simulink model "ctrl_TT"  (R2022b)
settings: Solver=FixedStepAuto  StartTime=0.0  StopTime=Tf  FixedStep=0.05  RelTol=1e-3
InitFcn:
  | run;
StopFcn:
  | save('testdata')
undefined symbols (not defined in the file): Ba_0, Bb, Bv_0, Bx_0, Cp, Cp_prime, d, dA_BP1, dA_BP2, dA_Hull, dA_PH, dA_Sail, dA_SProot, dA_X1a, dA_X1b, dA_X2a, dA_X2b, dA_X3a, dA_X3b, dA_X4a, dA_X4b, Ixx, Ixy, Ixz, Iyy, Iyz, Izz, Mb, n_BP1, n_BP2, n_Hull, n_PH, n_Sail, n_SProot, n_X2a, n_X2b, n_X3a, n_X4a, n_X4b, nt_BP1, nt_BP2, nt_Hull, nt_PH, nt_Sail, nt_SProot, nt_X1a, nt_X1b, nt_X2a, nt_X2b, nt_X3a, nt_X3b, nt_X4a, nt_X4b, Seastate, Tf, vt1_BP1, vt1_BP2, vt1_Hull, vt1_PH, vt1_Sail ... (+44)
libraries: simulink x8, sharedtransform x2, dspmathops x2
(part 3 of 5)

== system ctrl_TT/HDM/HDM B3/Z/ZdXi ==
  dX : Inport
  z : Inport  Port=2
  Demux6 : Demux  Outputs=5
  Mux : Mux  Inputs=5
  ZudX1 q+10 : Lookup_n-D  BreakpointsForDimension1=[-30 -20 -10 0 10 20 30]  BreakpointsForDimension2=[-35.0624 -15.3724 -13.8724]  BreakpointsForDimension3=[-35.0624 -15.3724 -13.8724]  Table=|  InternalRulePriority=Speed  RndMeth=Simplest
      | reshape([-0.003226964
      | -0.002116041
      | -0.001005119
      | 0.000105803
      | 0.001216725
      | 0.002327647
      | 0.003438569
      | -0.003036597
      | -0.001876165
      | -0.000715732
      | 0.0004447
      | 0.001605132
      | 0.002765565
      | 0.003925997
      | -0.003676642
      | -0.002490275
      | -0.001303908
      | -0.000117541
      | 0.001068826
      | 0.002255193
      | 0.00344156],[7,3])
      settings: InputPortMap=u0,u1
  ZudX1 q+6 : Lookup_n-D  BreakpointsForDimension1=[-30 -20 -10 0 10 20 30]  BreakpointsForDimension2=[-35.0624 -15.3724 -13.8724]  BreakpointsForDimension3=[-5.14444 -3.08666664 -1.54332]  Table=|  InternalRulePriority=Speed  RndMeth=Simplest
      | reshape([-0.001383757
      | -0.000911
      | -0.000438243
      | 3.45135E-05
      | 0.00050727
      | 0.000980027
      | 0.001452784
      | -0.001383757
      | -0.000911
      | -0.000438243
      | 3.45135E-05
      | 0.00050727
      | 0.000980027
      | 0.001452784
      | -0.001353354
      | -0.000887631
      | -0.000421908
      | 4.38143E-05
      | 0.000509537
      | 0.00097526
      | 0.001440982],[7,3])
      settings: InputPortMap=u0,u1
  ZudX1 q+7 : Lookup_n-D  BreakpointsForDimension1=[-30 -20 -10 0 10 20 30]  BreakpointsForDimension2=[-35.0624 -15.3724 -13.8724]  BreakpointsForDimension3=[-5.14444 -3.08666664 -1.54332]  Table=|  InternalRulePriority=Speed  RndMeth=Simplest
      | reshape([-0.001358511
      | -0.00091651
      | -0.000474508
      | -3.25062E-05
      | 0.000409495
      | 0.000851497
      | 0.001293499
      | -0.001303275
      | -0.00086798
      | -0.000432686
      | 2.60877E-06
      | 0.000437903
      | 0.000873198
      | 0.001308493
      | -0.001263287
      | -0.000836064
      | -0.00040884
      | 1.83841E-05
      | 0.000445608
      | 0.000872832
      | 0.001300056],[7,3])
      settings: InputPortMap=u0,u1
  ZudX1 q+8 : Lookup_n-D  BreakpointsForDimension1=[-30 -20 -10 0 10 20 30]  BreakpointsForDimension2=[-35.0624 -15.3724 -13.8724]  BreakpointsForDimension3=[-5.14444 -3.08666664 -1.54332]  Table=|  InternalRulePriority=Speed  RndMeth=Simplest
      | reshape([0.001309084
      | 0.000864124
      | 0.000419163
      | -2.5798E-05
      | -0.000470759
      | -0.000915719
      | -0.00136068
      | 0.001321953
      | 0.000882434
      | 0.000442915
      | 3.39516E-06
      | -0.000436124
      | -0.000875644
      | -0.001315163
      | 0.001313186
      | 0.000881448
      | 0.000449709
      | 1.79712E-05
      | -0.000413767
      | -0.000845505
      | -0.001277243],[7,3])
      settings: InputPortMap=u0,u1
  ZudX1 q+9 : Lookup_n-D  BreakpointsForDimension1=[-30 -20 -10 0 10 20 30]  BreakpointsForDimension2=[-35.0624 -15.3724 -13.8724]  BreakpointsForDimension3=[-5.14444 -3.08666664 -1.54332]  Table=|  InternalRulePriority=Speed  RndMeth=Simplest
      | reshape([0.001464336
      | 0.000977857
      | 0.000491377
      | 4.89775E-06
      | -0.000481582
      | -0.000968061
      | -0.00145454
      | 0.001455937
      | 0.00098192
      | 0.000507903
      | 3.38863E-05
      | -0.00044013
      | -0.000914147
      | -0.001388164
      | 0.001460604
      | 0.00098818
      | 0.000515756
      | 4.33325E-05
      | -0.000429091
      | -0.000901515
      | -0.001373939],[7,3])
      settings: InputPortMap=u0,u1
  ZdX : Outport
  wires:
  Demux6/3 -> ZudX1 q+8/1
  dX/1 -> Demux6/1
  Demux6/4 -> ZudX1 q+9/1
  Demux6/2 -> ZudX1 q+7/1
  Demux6/1 -> ZudX1 q+6/1
  Mux/1 -> ZdX/1
  Demux6/5 -> ZudX1 q+10/1
  z/1 -> ZudX1 q+6/2, ZudX1 q+7/2, ZudX1 q+8/2, ZudX1 q+10/2, ZudX1 q+9/2
  ZudX1 q+10/1 -> Mux/5
  ZudX1 q+6/1 -> Mux/1
  ZudX1 q+7/1 -> Mux/2
  ZudX1 q+8/1 -> Mux/3
  ZudX1 q+9/1 -> Mux/4

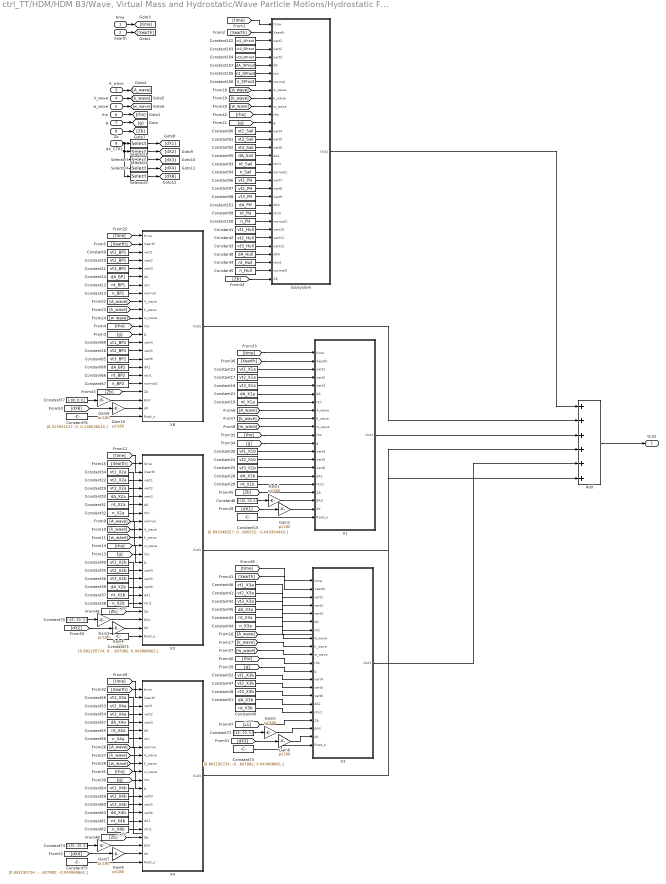
== system ctrl_TT/HDM/HDM B3/Wave, Virtual Mass and Hydrostatic/Wave Particle Motions/Hydrostatic Forces and Moments ==
  note: n_BP
  note: n_BP
  note: n_BP
  time : Inport
  Xearth : Inport  Port=2
  A_wave : Inport  Port=3
  k_wave : Inport  Port=4
  w_wave : Inport  Port=5
  rho : Inport  Port=6
  g : Inport  Port=7
  Zb : Inport  Port=8
  dX_CTRL : Inport  Port=9
  Add : Sum  Inputs=6
  Constant1 : Constant  Value=vt1_Hull
  Constant10 : Constant  Value=vt2_BP1
  Constant100 : Constant  Value=n_PH
  Constant101 : Constant  Value=dA_PH
  Constant102 : Constant  Value=vt1_SProot
  Constant103 : Constant  Value=vt2_SProot
  Constant104 : Constant  Value=vt3_SProot
  Constant105 : Constant  Value=nt_SProot
  Constant106 : Constant  Value=n_SProot
  Constant107 : Constant  Value=dA_SProot
  Constant11 : Constant  Value=vt3_BP1
  Constant12 : Constant  Value=nt_BP1
  Constant13 : Constant  Value=n_BP1
  Constant14 : Constant  Value=dA_BP1
  Constant15 : Constant  Value=|
      | [0.893348257;
      | 0.043600552;
      | -0.043394945;]
  Constant16 : Constant  Value=vt2_BP2
  Constant17 : Constant  Value=vt2_X1a
  Constant18 : Constant  Value=vt3_X1a
  Constant19 : Constant  Value=nt_X1a
  Constant2 : Constant  Value=vt2_Hull
  Constant21 : Constant  Value=dA_X1a
  Constant22 : Constant  Value=vt2_X2a
  Constant23 : Constant  Value=vt1_X1a
  Constant24 : Constant  Value=vt2_X1b
  Constant25 : Constant  Value=vt3_X1b
  Constant26 : Constant  Value=nt_X1b
  Constant28 : Constant  Value=dA_X1b
  Constant29 : Constant  Value=vt3_X2a
  Constant3 : Constant  Value=vt3_Hull
  Constant30 : Constant  Value=vt1_X1b
  Constant31 : Constant  Value=nt_X2a
  Constant32 : Constant  Value=n_X2a
  Constant33 : Constant  Value=dA_X2a
  Constant34 : Constant  Value=vt1_X2a
  Constant35 : Constant  Value=vt2_X2b
  Constant36 : Constant  Value=vt3_X2b
  Constant37 : Constant  Value=nt_X2b
  Constant38 : Constant  Value=n_X2b
  Constant39 : Constant  Value=dA_X2b
  Constant4 : Constant  Value=nt_Hull
  Constant40 : Constant  Value=vt1_X2b
  Constant41 : Constant  Value=vt2_X3a
  Constant42 : Constant  Value=vt3_X3a
  Constant43 : Constant  Value=nt_X3a
  Constant44 : Constant  Value=n_X3a
  Constant45 : Constant  Value=dA_X3a
  Constant46 : Constant  Value=vt1_X3a
  Constant47 : Constant  Value=vt2_X3b
  Constant48 : Constant  Value=vt3_X3b
  Constant49 : Constant  Value=nt_X3b
  Constant5 : Constant  Value=n_Hull
  Constant51 : Constant  Value=dA_X3b
  Constant52 : Constant  Value=vt1_X3b
  Constant53 : Constant  Value=vt2_X4a
  Constant54 : Constant  Value=vt3_X4a
  Constant55 : Constant  Value=nt_X4a
  Constant56 : Constant  Value=n_X4a
  Constant57 : Constant  Value=dA_X4a
  Constant58 : Constant  Value=vt1_X4a
  Constant59 : Constant  Value=vt2_X4b
  Constant6 : Constant  Value=[-135; -20; 0;]
  Constant60 : Constant  Value=vt3_X4b
  Constant61 : Constant  Value=nt_X4b
  Constant62 : Constant  Value=n_X4b
  Constant63 : Constant  Value=dA_X4b
  Constant64 : Constant  Value=vt1_X4b
  Constant65 : Constant  Value=vt3_BP2
  Constant66 : Constant  Value=nt_BP2
  Constant67 : Constant  Value=n_BP2
  Constant68 : Constant  Value=dA_BP2
  Constant69 : Constant  Value=vt1_BP2
  Constant70 : Constant  Value=[-45; -20; 0;]
  Constant71 : Constant  Value=|
      | [0.892195724;
      | 0.043607982;
      | 0.043868661;]
  Constant72 : Constant  Value=[45; -20; 0;]
  Constant73 : Constant  Value=|
      | [0.892195724;
      | -0.043607982;
      | 0.043868661;]
  Constant74 : Constant  Value=[135; -20; 0;]
  Constant75 : Constant  Value=|
      | [0.892195724;
      | -0.043607982;
      | -0.043868661;]
  Constant76 : Constant  Value=|
      | [0.313941517;
      | 0;
      | 0.138536015;]
  Constant77 : Constant  Value=[-90; 0; 0;]
  Constant8 : Constant  Value=dA_Hull
  Constant9 : Constant  Value=vt1_BP1
  Constant90 : Constant  Value=vt1_Sail
  Constant91 : Constant  Value=vt2_Sail
  Constant92 : Constant  Value=vt3_Sail
  Constant93 : Constant  Value=nt_Sail
  Constant94 : Constant  Value=n_Sail
  Constant95 : Constant  Value=dA_Sail
  Constant96 : Constant  Value=vt1_PH
  Constant97 : Constant  Value=vt2_PH
  Constant98 : Constant  Value=vt3_PH
  Constant99 : Constant  Value=nt_PH
  Gain{1..10} (10 alike) : Gain  Gain=pi/180
  Selector1 : Selector  InputPortWidth=5  IndexOptions=Index vector (dialog)  Indices=1  OutputSizes=1
  Selector2 : Selector  InputPortWidth=5  IndexOptions=Index vector (dialog)  Indices=2  OutputSizes=1
  Selector3 : Selector  InputPortWidth=5  IndexOptions=Index vector (dialog)  Indices=3  OutputSizes=1
  Selector4 : Selector  InputPortWidth=5  IndexOptions=Index vector (dialog)  Indices=4  OutputSizes=1
  Selector5 : Selector  InputPortWidth=5  IndexOptions=Index vector (dialog)  Indices=5  OutputSizes=1
  Subsystem : Subsystem
  X1 : Subsystem
  X2 : Subsystem
  X3 : Subsystem
  X4 : Subsystem
  XB : Subsystem
  Out1 : Outport
  wires:
  Subsystem/1(Out1) -> Add/1
  XB/1(Out1) -> Add/2
  X1/1(Out1) -> Add/3
  X2/1(Out1) -> Add/4
  X3/1(Out1) -> Add/5
  X4/1(Out1) -> Add/6
  Gain10/1 -> XB/22(dX)
  Constant76/1 -> XB/23(Root_o)
  [dXB] -> Gain10/1
  Gain9/1 -> XB/21(EAX)
  Constant77/1 -> Gain9/1
  Gain8/1 -> X4/21(dX)
  [dX4] -> Gain8/1
  Constant74/1 -> Gain7/1
  Gain7/1 -> X4/20(EAX)
  Constant75/1 -> X4/22(Root_o)
  Constant73/1 -> X3/21(Root_o)
  Gain6/1 -> X3/20(dX)
  Constant72/1 -> Gain5/1
  [dX3] -> Gain6/1
  Gain5/1 -> X3/19(EAX)
  Constant71/1 -> X2/22(Root_o)
  Gain4/1 -> X2/21(dX)
  [dX2] -> Gain4/1
  Gain3/1 -> X2/20(EAX)
  Constant70/1 -> Gain3/1
  Constant15/1 -> X1/21(Root_o)
  Gain2/1 -> X1/20(dX)
  [dX1] -> Gain2/1
  Selector5/1 -> [dXB]
  Selector4/1 -> [dX4]
  Selector3/1 -> [dX3]
  Selector2/1 -> [dX2]
  Selector1/1 -> [dX1]
  dX_CTRL/1 -> Selector1/1, Selector4/1, Selector5/1, Selector3/1, Selector2/1
  Gain1/1 -> X1/19(EAX)
  Constant6/1 -> Gain1/1
  Zb/1 -> [Zb]
  [A_wave] -> X3/8(A_wave)
  Constant5/1 -> Subsystem/31(normal3)
  Constant58/1 -> X4/3(vert1)
  Constant42/1 -> X3/5(vert3)
  [g] -> XB/13(g)
  Constant3/1 -> Subsystem/28(vert12)
  Constant103/1 -> Subsystem/4(vert2)
  Add/1 -> Out1/1
  [A_wave] -> Subsystem/9(A_wave)
  Constant10/1 -> XB/4(vert2)
  [time] -> X4/1(time)
  [k_wave] -> X4/10(k_wave)
  Constant38/1 -> ?
  Constant54/1 -> X4/5(vert3)
  Constant66/1 -> XB/18(ntri1)
  Constant2/1 -> Subsystem/27(vert11)
  Constant97/1 -> Subsystem/21(vert8)
  Constant64/1 -> X4/14(vert4)
  [Xearth] -> X4/2(Xearth)
  Constant29/1 -> X2/5(vert3)
  Constant36/1 -> X2/16(vert6)
  Constant96/1 -> Subsystem/20(vert7)
  Constant90/1 -> Subsystem/14(vert4)
  Constant21/1 -> X1/6(dA)
  [w_wave] -> X2/11(w_wave)
  Constant31/1 -> X2/7(ntri)
  Constant1/1 -> Subsystem/26(vert10)
  [time] -> X1/1(time)
  Constant91/1 -> Subsystem/15(vert5)
  [rho] -> X1/11(rho)
  [time] -> X2/1(time)
  Constant30/1 -> X1/13(vert4)
  Constant92/1 -> Subsystem/16(vert6)
  Constant100/1 -> Subsystem/25(normal2)
  [w_wave] -> X1/10(w_wave)
  [g] -> X3/12(g)
  Constant12/1 -> XB/7(ntri)
  Constant24/1 -> X1/14(vert5)
  Constant56/1 -> X4/8(normal)
  Constant26/1 -> X1/17(ntri1)
  [A_wave] -> XB/9(A_wave)
  Constant62/1 -> ?
  Constant9/1 -> XB/3(vert1)
  Constant23/1 -> X1/3(vert1)
  Constant46/1 -> X3/3(vert1)
  Constant68/1 -> XB/17(dA1)
  [k_wave] -> XB/10(k_wave)
  Constant17/1 -> X1/4(vert2)
  [A_wave] -> X2/9(A_wave)
  [k_wave] -> X3/9(k_wave)
  Constant43/1 -> X3/7(ntri)
  Constant69/1 -> XB/14(vert4)
  Constant13/1 -> XB/8(normal)
  Constant104/1 -> Subsystem/5(vert3)
  Constant65/1 -> XB/16(vert6)
  [Zb] -> Subsystem/32(Zb)
  Constant67/1 -> XB/19(normal1)
  Constant25/1 -> X1/15(vert6)
  [Xearth] -> X3/2(Xearth)
  Constant14/1 -> XB/6(dA)
  Constant52/1 -> X3/13(vert4)
  Constant51/1 -> X3/16(dA1)
  Constant59/1 -> X4/15(vert5)
  Constant4/1 -> Subsystem/30(ntri3)
  [rho] -> XB/12(rho)
  [time] -> XB/1(time)
  [Xearth] -> X2/2(Xearth)
  [w_wave] -> XB/11(w_wave)
  Constant53/1 -> X4/4(vert2)
  [k_wave] -> X1/9(k_wave)
  Constant44/1 -> ?
  [w_wave] -> X4/11(w_wave)
  Constant47/1 -> X3/14(vert5)
  Constant32/1 -> X2/8(normal)
  Constant39/1 -> X2/17(dA1)
  Constant35/1 -> X2/15(vert5)
  [g] -> X1/12(g)
  Constant18/1 -> X1/5(vert3)
  Constant40/1 -> X2/14(vert4)
  Constant45/1 -> X3/6(dA)
  Constant55/1 -> X4/7(ntri)
  [rho] -> X3/11(rho)
  [rho] -> X2/12(rho)
  [Xearth] -> XB/2(Xearth)
  Constant49/1 -> X3/17(ntri1)
  Constant22/1 -> X2/4(vert2)
  [k_wave] -> X2/10(k_wave)
  Constant41/1 -> X3/4(vert2)
  [A_wave] -> X1/8(A_wave)
  Constant63/1 -> X4/17(dA1)
  Constant34/1 -> X2/3(vert1)
  Constant11/1 -> XB/5(vert3)
  [g] -> X4/13(g)
  Constant105/1 -> Subsystem/7(ntri)
  Constant107/1 -> Subsystem/6(dA)
  [Xearth] -> Subsystem/2(Xearth)
  Constant106/1 -> Subsystem/8(normal)
  Constant102/1 -> Subsystem/3(vert1)
  [g] -> Subsystem/13(g)
  Constant19/1 -> X1/7(ntri)
  [k_wave] -> Subsystem/10(k_wave)
  Constant60/1 -> X4/16(vert6)
  [rho] -> Subsystem/12(rho)
  Constant48/1 -> X3/15(vert6)
  [time] -> Subsystem/1(time)
  [rho] -> X4/12(rho)
  Constant33/1 -> X2/6(dA)
  [A_wave] -> X4/9(A_wave)
  Constant95/1 -> Subsystem/17(dA1)
  Constant8/1 -> Subsystem/29(dA3)
  [w_wave] -> X3/10(w_wave)
  Constant28/1 -> X1/16(dA1)
  [g] -> X2/13(g)
  Constant93/1 -> Subsystem/18(ntri1)
  [w_wave] -> Subsystem/11(w_wave)
  [Xearth] -> X1/2(Xearth)
  [time] -> X3/1(time)
  [Zb] -> XB/20(Zb)
  Constant37/1 -> X2/18(ntri1)
  Constant99/1 -> Subsystem/24(ntri2)
  Constant98/1 -> Subsystem/22(vert9)
  [Zb] -> X2/19(Zb)
  [Zb] -> X1/18(Zb)
  Constant16/1 -> XB/15(vert5)
  Constant101/1 -> Subsystem/23(dA2)
  [Zb] -> X3/18(Zb)
  [Zb] -> X4/19(Zb)
  Constant57/1 -> X4/6(dA)
  Constant61/1 -> X4/18(ntri1)
  Constant94/1 -> Subsystem/19(normal1)
  g/1 -> [g]
  rho/1 -> [rho]
  w_wave/1 -> [w_wave]
  k_wave/1 -> [k_wave]
  A_wave/1 -> [A_wave]
  Xearth/1 -> [Xearth]
  time/1 -> [time]

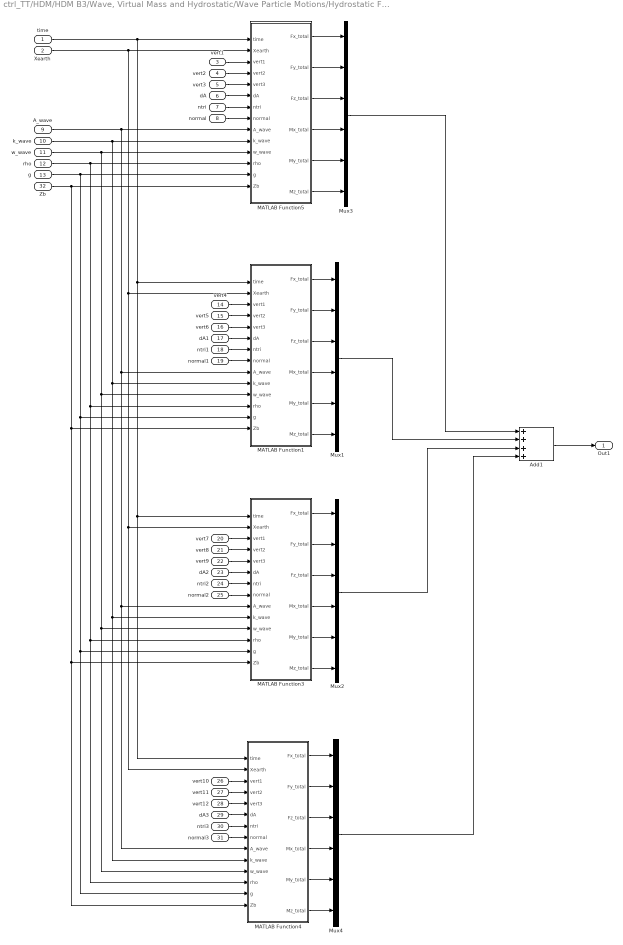
== system ctrl_TT/HDM/HDM B3/Wave, Virtual Mass and Hydrostatic/Wave Particle Motions/Hydrostatic Forces and Moments/Subsystem ==
  time : Inport
  Xearth : Inport  Port=2
  vert1 : Inport  Port=3
  vert2 : Inport  Port=4
  vert3 : Inport  Port=5
  dA : Inport  Port=6
  ntri : Inport  Port=7
  normal : Inport  Port=8
  A_wave : Inport  Port=9
  k_wave : Inport  Port=10
  w_wave : Inport  Port=11
  rho : Inport  Port=12
  g : Inport  Port=13
  vert4 : Inport  Port=14
  vert5 : Inport  Port=15
  vert6 : Inport  Port=16
  dA1 : Inport  Port=17
  ntri1 : Inport  Port=18
  normal1 : Inport  Port=19
  vert7 : Inport  Port=20
  vert8 : Inport  Port=21
  vert9 : Inport  Port=22
  dA2 : Inport  Port=23
  ntri2 : Inport  Port=24
  normal2 : Inport  Port=25
  vert10 : Inport  Port=26
  vert11 : Inport  Port=27
  vert12 : Inport  Port=28
  dA3 : Inport  Port=29
  ntri3 : Inport  Port=30
  normal3 : Inport  Port=31
  Zb : Inport  Port=32
  Add1 : Sum  Inputs=4
  MATLAB Function1 : MATLAB Function  TreatAsAtomicUnit=on
  MATLAB Function3 : MATLAB Function  TreatAsAtomicUnit=on
  MATLAB Function4 : MATLAB Function  TreatAsAtomicUnit=on
  MATLAB Function5 : MATLAB Function  TreatAsAtomicUnit=on
  Mux{1..4} (4 alike) : Mux  Inputs=6
  Out1 : Outport
  wires:
  Mux4/1 -> Add1/4
  MATLAB Function4/5(My_total) -> Mux4/5
  MATLAB Function4/4(Mx_total) -> Mux4/4
  MATLAB Function4/3(Fz_total) -> Mux4/3
  MATLAB Function4/2(Fy_total) -> Mux4/2
  MATLAB Function4/1(Fx_total) -> Mux4/1
  MATLAB Function4/6(Mz_total) -> Mux4/6
  MATLAB Function3/6(Mz_total) -> Mux2/6
  MATLAB Function3/1(Fx_total) -> Mux2/1
  MATLAB Function3/2(Fy_total) -> Mux2/2
  MATLAB Function3/3(Fz_total) -> Mux2/3
  MATLAB Function3/4(Mx_total) -> Mux2/4
  MATLAB Function3/5(My_total) -> Mux2/5
  MATLAB Function1/5(My_total) -> Mux1/5
  MATLAB Function1/4(Mx_total) -> Mux1/4
  MATLAB Function1/3(Fz_total) -> Mux1/3
  MATLAB Function1/2(Fy_total) -> Mux1/2
  MATLAB Function1/1(Fx_total) -> Mux1/1
  Mux1/1 -> Add1/2
  MATLAB Function1/6(Mz_total) -> Mux1/6
  Mux2/1 -> Add1/3
  Zb/1 -> MATLAB Function4/14(Zb), MATLAB Function3/14(Zb), MATLAB Function1/14(Zb), MATLAB Function5/14(Zb)
  vert8/1 -> MATLAB Function3/4(vert2)
  vert1/1 -> MATLAB Function5/3(vert1)
  vert10/1 -> MATLAB Function4/3(vert1)
  dA1/1 -> MATLAB Function1/6(dA)
  normal2/1 -> MATLAB Function3/8(normal)
  vert3/1 -> MATLAB Function5/5(vert3)
  vert6/1 -> MATLAB Function1/5(vert3)
  Add1/1 -> Out1/1
  vert2/1 -> MATLAB Function5/4(vert2)
  dA3/1 -> MATLAB Function4/6(dA)
  ntri3/1 -> MATLAB Function4/7(ntri)
  ntri2/1 -> MATLAB Function3/7(ntri)
  vert11/1 -> MATLAB Function4/4(vert2)
  MATLAB Function5/6(Mz_total) -> Mux3/6
  dA/1 -> MATLAB Function5/6(dA)
  normal/1 -> MATLAB Function5/8(normal)
  vert9/1 -> MATLAB Function3/5(vert3)
  vert4/1 -> MATLAB Function1/3(vert1)
  normal3/1 -> MATLAB Function4/8(normal)
  vert12/1 -> MATLAB Function4/5(vert3)
  MATLAB Function5/1(Fx_total) -> Mux3/1
  dA2/1 -> MATLAB Function3/6(dA)
  g/1 -> MATLAB Function3/13(g), MATLAB Function4/13(g), MATLAB Function1/13(g), MATLAB Function5/13(g)
  ntri/1 -> MATLAB Function5/7(ntri)
  MATLAB Function5/2(Fy_total) -> Mux3/2
  w_wave/1 -> MATLAB Function3/11(w_wave), MATLAB Function4/11(w_wave), MATLAB Function1/11(w_wave), MATLAB Function5/11(w_wave)
  k_wave/1 -> MATLAB Function3/10(k_wave), MATLAB Function4/10(k_wave), MATLAB Function1/10(k_wave), MATLAB Function5/10(k_wave)
  MATLAB Function5/3(Fz_total) -> Mux3/3
  A_wave/1 -> MATLAB Function3/9(A_wave), MATLAB Function4/9(A_wave), MATLAB Function1/9(A_wave), MATLAB Function5/9(A_wave)
  normal1/1 -> MATLAB Function1/8(normal)
  Mux3/1 -> Add1/1
  MATLAB Function5/4(Mx_total) -> Mux3/4
  vert7/1 -> MATLAB Function3/3(vert1)
  Xearth/1 -> MATLAB Function1/2(Xearth), MATLAB Function3/2(Xearth), MATLAB Function4/2(Xearth), MATLAB Function5/2(Xearth)
  time/1 -> MATLAB Function3/1(time), MATLAB Function4/1(time), MATLAB Function1/1(time), MATLAB Function5/1(time)
  MATLAB Function5/5(My_total) -> Mux3/5
  vert5/1 -> MATLAB Function1/4(vert2)
  rho/1 -> MATLAB Function3/12(rho), MATLAB Function4/12(rho), MATLAB Function1/12(rho), MATLAB Function5/12(rho)
  ntri1/1 -> MATLAB Function1/7(ntri)

== system ctrl_TT/HDM/HDM B3/Wave, Virtual Mass and Hydrostatic/Wave Particle Motions/Hydrostatic Forces and Moments/X1 ==
  time : Inport
  Xearth : Inport  Port=2
  vert1 : Inport  Port=3
  vert2 : Inport  Port=4
  vert3 : Inport  Port=5
  dA : Inport  Port=6
  ntri : Inport  Port=7
  A_wave : Inport  Port=8
  k_wave : Inport  Port=9
  w_wave : Inport  Port=10
  rho : Inport  Port=11
  g : Inport  Port=12
  vert4 : Inport  Port=13
  vert5 : Inport  Port=14
  vert6 : Inport  Port=15
  dA1 : Inport  Port=16
  ntri1 : Inport  Port=17
  Zb : Inport  Port=18
  EAX : Inport  Port=19
  dX : Inport  Port=20
  Root_o : Inport  Port=21
  Add1 : Sum
  CG : Constant  Value=[32.3114; 0; 0;]
  MATLAB Function1 : MATLAB Function  TreatAsAtomicUnit=on
  MATLAB Function4 : MATLAB Function  TreatAsAtomicUnit=on
  Mux1 : Mux  Inputs=6
  Mux2 : Mux  Inputs=6
  Out1 : Outport
  wires:
  MATLAB Function1/6(Mz_total) -> Mux1/6
  MATLAB Function1/5(My_total) -> Mux1/5
  CG/1 -> MATLAB Function4/17(xcg), MATLAB Function1/17(xcg)
  Root_o/1 -> MATLAB Function4/16(origin), MATLAB Function1/16(origin)
  dX/1 -> MATLAB Function1/15(dX), MATLAB Function4/15(dX)
  EAX/1 -> MATLAB Function4/14(EAX), MATLAB Function1/14(EAX)
  MATLAB Function4/3(Fz_total) -> Mux2/3
  MATLAB Function4/4(Mx_total) -> Mux2/4
  w_wave/1 -> MATLAB Function4/10(w_wave), MATLAB Function1/10(w_wave)
  MATLAB Function1/2(Fy_total) -> Mux1/2
  Xearth/1 -> MATLAB Function1/2(Xearth), MATLAB Function4/2(Xearth)
  rho/1 -> MATLAB Function4/11(rho), MATLAB Function1/11(rho)
  A_wave/1 -> MATLAB Function4/8(A_wave), MATLAB Function1/8(A_wave)
  MATLAB Function1/4(Mx_total) -> Mux1/4
  MATLAB Function4/1(Fx_total) -> Mux2/1
  MATLAB Function1/1(Fx_total) -> Mux1/1
  Add1/1 -> Out1/1
  MATLAB Function1/3(Fz_total) -> Mux1/3
  MATLAB Function4/5(My_total) -> Mux2/5
  dA/1 -> MATLAB Function4/6(dA)
  k_wave/1 -> MATLAB Function1/9(k_wave), MATLAB Function4/9(k_wave)
  g/1 -> MATLAB Function4/12(g), MATLAB Function1/12(g)
  MATLAB Function4/6(Mz_total) -> Mux2/6
  MATLAB Function4/2(Fy_total) -> Mux2/2
  Mux2/1 -> Add1/1
  vert3/1 -> MATLAB Function4/5(vert3)
  Mux1/1 -> Add1/2
  vert1/1 -> MATLAB Function4/3(vert1)
  time/1 -> MATLAB Function1/1(time), MATLAB Function4/1(time)
  ntri/1 -> MATLAB Function4/7(ntri)
  vert2/1 -> MATLAB Function4/4(vert2)
  Zb/1 -> MATLAB Function4/13(Zb), MATLAB Function1/13(Zb)
  vert4/1 -> MATLAB Function1/3(vert1)
  vert5/1 -> MATLAB Function1/4(vert2)
  vert6/1 -> MATLAB Function1/5(vert3)
  dA1/1 -> MATLAB Function1/6(dA)
  ntri1/1 -> MATLAB Function1/7(ntri)

== system ctrl_TT/HDM/HDM B3/Wave, Virtual Mass and Hydrostatic/Wave Particle Motions/Hydrostatic Forces and Moments/X2 ==
  time : Inport
  Xearth : Inport  Port=2
  vert1 : Inport  Port=3
  vert2 : Inport  Port=4
  vert3 : Inport  Port=5
  dA : Inport  Port=6
  ntri : Inport  Port=7
  normal : Inport  Port=8
  A_wave : Inport  Port=9
  k_wave : Inport  Port=10
  w_wave : Inport  Port=11
  rho : Inport  Port=12
  g : Inport  Port=13
  vert4 : Inport  Port=14
  vert5 : Inport  Port=15
  vert6 : Inport  Port=16
  dA1 : Inport  Port=17
  ntri1 : Inport  Port=18
  Zb : Inport  Port=19
  EAX : Inport  Port=20
  dX : Inport  Port=21
  Root_o : Inport  Port=22
  Add1 : Sum
  CG : Constant  Value=[32.3114; 0; 0;]
  MATLAB Function1 : MATLAB Function  TreatAsAtomicUnit=on
  MATLAB Function4 : MATLAB Function  TreatAsAtomicUnit=on
  Mux1 : Mux  Inputs=6
  Mux2 : Mux  Inputs=6
  Out1 : Outport
  wires:
  ntri1/1 -> MATLAB Function1/7(ntri)
  dA1/1 -> MATLAB Function1/6(dA)
  vert6/1 -> MATLAB Function1/5(vert3)
  vert5/1 -> MATLAB Function1/4(vert2)
  vert4/1 -> MATLAB Function1/3(vert1)
  Zb/1 -> MATLAB Function4/13(Zb), MATLAB Function1/13(Zb)
  vert2/1 -> MATLAB Function4/4(vert2)
  ntri/1 -> MATLAB Function4/7(ntri)
  normal/1 -> ?
  time/1 -> MATLAB Function4/1(time), MATLAB Function1/1(time)
  vert1/1 -> MATLAB Function4/3(vert1)
  Mux1/1 -> Add1/2
  vert3/1 -> MATLAB Function4/5(vert3)
  Mux2/1 -> Add1/1
  MATLAB Function4/2(Fy_total) -> Mux2/2
  MATLAB Function4/6(Mz_total) -> Mux2/6
  g/1 -> MATLAB Function4/12(g), MATLAB Function1/12(g)
  k_wave/1 -> MATLAB Function4/9(k_wave), MATLAB Function1/9(k_wave)
  dA/1 -> MATLAB Function4/6(dA)
  MATLAB Function4/5(My_total) -> Mux2/5
  MATLAB Function1/3(Fz_total) -> Mux1/3
  Add1/1 -> Out1/1
  MATLAB Function1/1(Fx_total) -> Mux1/1
  MATLAB Function4/1(Fx_total) -> Mux2/1
  MATLAB Function1/4(Mx_total) -> Mux1/4
  A_wave/1 -> MATLAB Function4/8(A_wave), MATLAB Function1/8(A_wave)
  rho/1 -> MATLAB Function4/11(rho), MATLAB Function1/11(rho)
  Xearth/1 -> MATLAB Function4/2(Xearth), MATLAB Function1/2(Xearth)
  MATLAB Function1/2(Fy_total) -> Mux1/2
  w_wave/1 -> MATLAB Function4/10(w_wave), MATLAB Function1/10(w_wave)
  MATLAB Function4/4(Mx_total) -> Mux2/4
  MATLAB Function4/3(Fz_total) -> Mux2/3
  EAX/1 -> MATLAB Function4/14(EAX), MATLAB Function1/14(EAX)
  dX/1 -> MATLAB Function4/15(dX), MATLAB Function1/15(dX)
  Root_o/1 -> MATLAB Function4/16(origin), MATLAB Function1/16(origin)
  CG/1 -> MATLAB Function4/17(xcg), MATLAB Function1/17(xcg)
  MATLAB Function1/5(My_total) -> Mux1/5
  MATLAB Function1/6(Mz_total) -> Mux1/6

== system ctrl_TT/HDM/HDM B3/Wave, Virtual Mass and Hydrostatic/Wave Particle Motions/Hydrostatic Forces and Moments/X3 ==
  time : Inport
  Xearth : Inport  Port=2
  vert1 : Inport  Port=3
  vert2 : Inport  Port=4
  vert3 : Inport  Port=5
  dA : Inport  Port=6
  ntri : Inport  Port=7
  A_wave : Inport  Port=8
  k_wave : Inport  Port=9
  w_wave : Inport  Port=10
  rho : Inport  Port=11
  g : Inport  Port=12
  vert4 : Inport  Port=13
  vert5 : Inport  Port=14
  vert6 : Inport  Port=15
  dA1 : Inport  Port=16
  ntri1 : Inport  Port=17
  Zb : Inport  Port=18
  EAX : Inport  Port=19
  dX : Inport  Port=20
  Root_o : Inport  Port=21
  Add1 : Sum
  CG : Constant  Value=[32.3114; 0; 0;]
  MATLAB Function1 : MATLAB Function  TreatAsAtomicUnit=on
  MATLAB Function4 : MATLAB Function  TreatAsAtomicUnit=on
  Mux1 : Mux  Inputs=6
  Mux2 : Mux  Inputs=6
  Out1 : Outport
  wires:
  MATLAB Function1/6(Mz_total) -> Mux1/6
  MATLAB Function1/5(My_total) -> Mux1/5
  CG/1 -> MATLAB Function1/17(xcg), MATLAB Function4/17(xcg)
  Root_o/1 -> MATLAB Function1/16(origin), MATLAB Function4/16(origin)
  dX/1 -> MATLAB Function1/15(dX), MATLAB Function4/15(dX)
  EAX/1 -> MATLAB Function1/14(EAX), MATLAB Function4/14(EAX)
  MATLAB Function4/3(Fz_total) -> Mux2/3
  MATLAB Function4/4(Mx_total) -> Mux2/4
  w_wave/1 -> MATLAB Function1/10(w_wave), MATLAB Function4/10(w_wave)
  MATLAB Function1/2(Fy_total) -> Mux1/2
  Xearth/1 -> MATLAB Function1/2(Xearth), MATLAB Function4/2(Xearth)
  rho/1 -> MATLAB Function1/11(rho), MATLAB Function4/11(rho)
  A_wave/1 -> MATLAB Function1/8(A_wave), MATLAB Function4/8(A_wave)
  MATLAB Function1/4(Mx_total) -> Mux1/4
  MATLAB Function4/1(Fx_total) -> Mux2/1
  MATLAB Function1/1(Fx_total) -> Mux1/1
  Add1/1 -> Out1/1
  MATLAB Function1/3(Fz_total) -> Mux1/3
  MATLAB Function4/5(My_total) -> Mux2/5
  dA/1 -> MATLAB Function4/6(dA)
  k_wave/1 -> MATLAB Function1/9(k_wave), MATLAB Function4/9(k_wave)
  g/1 -> MATLAB Function1/12(g), MATLAB Function4/12(g)
  MATLAB Function4/6(Mz_total) -> Mux2/6
  MATLAB Function4/2(Fy_total) -> Mux2/2
  Mux2/1 -> Add1/1
  vert3/1 -> MATLAB Function4/5(vert3)
  Mux1/1 -> Add1/2
  vert1/1 -> MATLAB Function4/3(vert1)
  time/1 -> MATLAB Function1/1(time), MATLAB Function4/1(time)
  ntri/1 -> MATLAB Function4/7(ntri)
  vert2/1 -> MATLAB Function4/4(vert2)
  Zb/1 -> MATLAB Function1/13(Zb), MATLAB Function4/13(Zb)
  vert4/1 -> MATLAB Function1/3(vert1)
  vert5/1 -> MATLAB Function1/4(vert2)
  vert6/1 -> MATLAB Function1/5(vert3)
  dA1/1 -> MATLAB Function1/6(dA)
  ntri1/1 -> MATLAB Function1/7(ntri)

== system ctrl_TT/HDM/HDM B3/Wave, Virtual Mass and Hydrostatic/Wave Particle Motions/Hydrostatic Forces and Moments/X4 ==
  time : Inport
  Xearth : Inport  Port=2
  vert1 : Inport  Port=3
  vert2 : Inport  Port=4
  vert3 : Inport  Port=5
  dA : Inport  Port=6
  ntri : Inport  Port=7
  normal : Inport  Port=8
  A_wave : Inport  Port=9
  k_wave : Inport  Port=10
  w_wave : Inport  Port=11
  rho : Inport  Port=12
  g : Inport  Port=13
  vert4 : Inport  Port=14
  vert5 : Inport  Port=15
  vert6 : Inport  Port=16
  dA1 : Inport  Port=17
  ntri1 : Inport  Port=18
  Zb : Inport  Port=19
  EAX : Inport  Port=20
  dX : Inport  Port=21
  Root_o : Inport  Port=22
  Add1 : Sum
  CG : Constant  Value=[32.3114; 0; 0;]
  MATLAB Function1 : MATLAB Function  TreatAsAtomicUnit=on
  MATLAB Function4 : MATLAB Function  TreatAsAtomicUnit=on
  Mux1 : Mux  Inputs=6
  Mux2 : Mux  Inputs=6
  Out1 : Outport
  wires:
  ntri1/1 -> MATLAB Function1/7(ntri)
  dA1/1 -> MATLAB Function1/6(dA)
  vert6/1 -> MATLAB Function1/5(vert3)
  vert5/1 -> MATLAB Function1/4(vert2)
  vert4/1 -> MATLAB Function1/3(vert1)
  Zb/1 -> MATLAB Function4/13(Zb), MATLAB Function1/13(Zb)
  vert2/1 -> MATLAB Function4/4(vert2)
  ntri/1 -> MATLAB Function4/7(ntri)
  normal/1 -> ?
  time/1 -> MATLAB Function4/1(time), MATLAB Function1/1(time)
  vert1/1 -> MATLAB Function4/3(vert1)
  Mux1/1 -> Add1/2
  vert3/1 -> MATLAB Function4/5(vert3)
  Mux2/1 -> Add1/1
  MATLAB Function4/2(Fy_total) -> Mux2/2
  MATLAB Function4/6(Mz_total) -> Mux2/6
  g/1 -> MATLAB Function4/12(g), MATLAB Function1/12(g)
  k_wave/1 -> MATLAB Function4/9(k_wave), MATLAB Function1/9(k_wave)
  dA/1 -> MATLAB Function4/6(dA)
  MATLAB Function4/5(My_total) -> Mux2/5
  MATLAB Function1/3(Fz_total) -> Mux1/3
  Add1/1 -> Out1/1
  MATLAB Function1/1(Fx_total) -> Mux1/1
  MATLAB Function4/1(Fx_total) -> Mux2/1
  MATLAB Function1/4(Mx_total) -> Mux1/4
  A_wave/1 -> MATLAB Function4/8(A_wave), MATLAB Function1/8(A_wave)
  rho/1 -> MATLAB Function1/11(rho), MATLAB Function4/11(rho)
  Xearth/1 -> MATLAB Function4/2(Xearth), MATLAB Function1/2(Xearth)
  MATLAB Function1/2(Fy_total) -> Mux1/2
  w_wave/1 -> MATLAB Function4/10(w_wave), MATLAB Function1/10(w_wave)
  MATLAB Function4/4(Mx_total) -> Mux2/4
  MATLAB Function4/3(Fz_total) -> Mux2/3
  EAX/1 -> MATLAB Function4/14(EAX), MATLAB Function1/14(EAX)
  dX/1 -> MATLAB Function4/15(dX), MATLAB Function1/15(dX)
  Root_o/1 -> MATLAB Function4/16(origin), MATLAB Function1/16(origin)
  CG/1 -> MATLAB Function4/17(xcg), MATLAB Function1/17(xcg)
  MATLAB Function1/5(My_total) -> Mux1/5
  MATLAB Function1/6(Mz_total) -> Mux1/6

== system ctrl_TT/HDM/HDM B3/Wave, Virtual Mass and Hydrostatic/Wave Particle Motions/Hydrostatic Forces and Moments/XB ==
  time : Inport
  Xearth : Inport  Port=2
  vert1 : Inport  Port=3
  vert2 : Inport  Port=4
  vert3 : Inport  Port=5
  dA : Inport  Port=6
  ntri : Inport  Port=7
  normal : Inport  Port=8
  A_wave : Inport  Port=9
  k_wave : Inport  Port=10
  w_wave : Inport  Port=11
  rho : Inport  Port=12
  g : Inport  Port=13
  vert4 : Inport  Port=14
  vert5 : Inport  Port=15
  vert6 : Inport  Port=16
  dA1 : Inport  Port=17
  ntri1 : Inport  Port=18
  normal1 : Inport  Port=19
  Zb : Inport  Port=20
  EAX : Inport  Port=21
  dX : Inport  Port=22
  Root_o : Inport  Port=23
  Add1 : Sum
  CG : Constant  Value=[32.3114; 0; 0;]
  MATLAB Function1 : MATLAB Function  TreatAsAtomicUnit=on
  MATLAB Function4 : MATLAB Function  TreatAsAtomicUnit=on
  Mux1 : Mux  Inputs=6
  Mux2 : Mux  Inputs=6
  Out1 : Outport
  wires:
  normal1/1 -> ?
  ntri1/1 -> MATLAB Function1/7(ntri)
  dA1/1 -> MATLAB Function1/6(dA)
  vert6/1 -> MATLAB Function1/5(vert3)
  vert5/1 -> MATLAB Function1/4(vert2)
  vert4/1 -> MATLAB Function1/3(vert1)
  Zb/1 -> MATLAB Function4/13(Zb), MATLAB Function1/13(Zb)
  vert2/1 -> MATLAB Function4/4(vert2)
  ntri/1 -> MATLAB Function4/7(ntri)
  normal/1 -> ?
  time/1 -> MATLAB Function4/1(time), MATLAB Function1/1(time)
  vert1/1 -> MATLAB Function4/3(vert1)
  Mux1/1 -> Add1/2
  vert3/1 -> MATLAB Function4/5(vert3)
  Mux2/1 -> Add1/1
  MATLAB Function4/2(Fy_total) -> Mux2/2
  MATLAB Function4/6(Mz_total) -> Mux2/6
  g/1 -> MATLAB Function4/12(g), MATLAB Function1/12(g)
  k_wave/1 -> MATLAB Function4/9(k_wave), MATLAB Function1/9(k_wave)
  dA/1 -> MATLAB Function4/6(dA)
  MATLAB Function4/5(My_total) -> Mux2/5
  MATLAB Function1/3(Fz_total) -> Mux1/3
  Add1/1 -> Out1/1
  MATLAB Function1/1(Fx_total) -> Mux1/1
  MATLAB Function4/1(Fx_total) -> Mux2/1
  MATLAB Function1/4(Mx_total) -> Mux1/4
  A_wave/1 -> MATLAB Function4/8(A_wave), MATLAB Function1/8(A_wave)
  rho/1 -> MATLAB Function4/11(rho), MATLAB Function1/11(rho)
  Xearth/1 -> MATLAB Function4/2(Xearth), MATLAB Function1/2(Xearth)
  MATLAB Function1/2(Fy_total) -> Mux1/2
  w_wave/1 -> MATLAB Function4/10(w_wave), MATLAB Function1/10(w_wave)
  MATLAB Function4/4(Mx_total) -> Mux2/4
  MATLAB Function4/3(Fz_total) -> Mux2/3
  EAX/1 -> MATLAB Function4/14(EAX), MATLAB Function1/14(EAX)
  dX/1 -> MATLAB Function4/15(dX), MATLAB Function1/15(dX)
  Root_o/1 -> MATLAB Function4/16(origin), MATLAB Function1/16(origin)
  CG/1 -> MATLAB Function4/17(xcg), MATLAB Function1/17(xcg)
  MATLAB Function1/5(My_total) -> Mux1/5
  MATLAB Function1/6(Mz_total) -> Mux1/6

== matlab function ctrl_TT/Controller/Subsystem1/MATLAB Function ==
  data: u input; y output
function y = R3(u)

y = [u(1,1) u(1,2) 0; u(2,1) u(2,2) 0; 0 0 1];

== matlab function ctrl_TT/Controller/MATLAB Function2 ==
  data: time input; pd output; pdp output; Cp_prime parameter; Cp parameter; Tf parameter
function [pd, pdp] = fcn(time, Cp_prime, Cp, Tf)




pd = BernsteinPoly(Cp,time,0,Tf);
pdp = BernsteinPoly(Cp_prime,time,0,Tf);

% pd = [gamma; gamma/2 ; -50];
% 
% 
% pdp = [1 ; 1/2; 0];

end










function  poly_t  = BernsteinPoly(Cp,t,t0,tf)

% INPUTS:
% Cp is a matrix n by N+1 (n: dimension of polynomial, N: order of polynomial) 
% t is a time vector
% OUTPUT:
% poly_t: n-dimensional polynomial evaluated at each time t

% if t is a scalar, it returns the value of Bernstein Poly at t in [t0,tf]
% if t0 and tf are not provided, it returns the value of Bernstein Poly at t in [0,1]

% Written by: Venanzio Cichella       

%%%%%%%%%%%%%%%%%%%%%%%%%%%%%%%%%%%%%%%%%%%%%%

coder.extrinsic('exist')

[~, N] = size(Cp);
N = N-1;


% if length(t) > 1
%     B = BernsteinMatrix_a2b(N,t)';
%     poly_t = Cp*B;
% else
%     if ~exist('t0','var')
%         B = BernsteinMatrix_a2b(N,t)';
%         poly_t = Cp*B;
%     else
%         B = BernsteinMatrix_a2b(N,t,t0,tf)';
%         poly_t = Cp*B;
%     end
% end
B = BernsteinMatrix_a2b(N,t,t0,tf)';
poly_t = Cp*B;


end










function b = BernsteinMatrix_a2b(N, t, tmin, tmax)

% Inputs: order N, time vector t = [t0 ... tm], no need for tmin and tmax.
% Output: b = [b0N(t0) b1N(t0) ... bNN(t0);
%              b0N(t1) b1N(t1) ... bNN(t1);
%              ...
%              b0N(tm) b1N(tm) ... bNN(tm);
% Use: If Cp is a row vector of N+1 control points,
%       the Nth order Bezier curve is given by xN=Cp*b';
% This function is used in BernsteinPoly

% Alternatively
% Inputs: order n, scalar time t', tmin and tmax
% Output: b = [b0n(t') b1n(t') ... bnn(t')]
% Use: If Cp is a row vector of N+1 control points,
%       the Nth order Bezier curve evaluated at t' is given by xn=Cp*b';
% Comment: This is more efficient but not as robust as de Casteljau
%           It works best for low-order curves

% Written by: Venanzio Cichella       

%%%%%%%%%%%%%%%%%%%%%%%%%%%%%%%%%%%%%%%%%%%%%%

if length(t) > 1
    tmax = t(length(t));
    tmin = t(1);
end
%coder.extrinsic('exist')
%if ~exist('tmin','var')
%    tmin = 0; tmax = 1;
%end



% compute B(j+1) = binomial(n, j), j = 0..n
t = t';
B = ones(N+1, 1); 
for j = 1:ceil(N/2)
  B(j+1) = B(j)*(N+1-j)/j;
  B(N+1-j) = B(j+1);
end
% compute T(i, j) = (t(i)-tmin)^j, TT(i, j) = (tmax-t(i))^(N-j)
T = ones(length(t), N+1);
TT = ones(length(t), N+1);
% turn a row t into a column t so that 
% we can do diag(t)*T(:,j) by t.*T(:,j)
tp = reshape(t, length(t), 1)-tmin;
ttp = tmax - t;
% Compute binomial(N, j)*(t(i)-tmin)^j*(tmax-t(i))^(N-j)
for j = 1:N 
  T(:, j+1) = tp .* T(:, j); 
  T(:, j) = T(:, j) .* B(j);
 TT(:,N+1-j) = ttp .* TT(:,N+2-j);
end

% Compute binomial(N, j)*(t(i)-tmin)^j*(tmax-t(i))^(N-j)/((tmax-tmin)^N)
b =  T.*TT./((tmax-tmin)^N);

end

== matlab function ctrl_TT/Controller/Subsystem1/Subsystem2/MATLAB Function ==
  data: a input; y output; b input
function y = fcn(a,b)

%y = [a,b,0;-b,a,0;0,0,1];
y = [a,b;-b,a];

== matlab function ctrl_TT/Controller/Marin PID ==
  settings: updateMethod=DISCRETE
  data: z_ref input; psi_ref input; Bv input; Bx input; dX output; Ts parameter
function dX   = fcn(z_ref,psi_ref,Bv,Bx,Ts)

persistent zerr_prev zerr_int_prev thetaerr_prev thetaerr_int_prev psierr_prev psierr_int_prev

%% Initialize
if isempty(zerr_prev)
        zerr_prev = 0;
        zerr_int_prev = 0;
        thetaerr_prev = 0;
        thetaerr_int_prev = 0;
        psierr_prev = 0;
        psierr_int_prev = 0;
end


%% Variables for feedback
x = Bx(1); y = Bx(2); z = Bx(3); phi = Bx(4); theta = Bx(5); psi = Bx(6);
p = [x;y;z];
uN = Bv(1); vN = Bv(2); wN = Bv(3); pB = Bv(4); qB=Bv(5); rB = Bv(6);
uB = -uN; vB = -vN; wB = wN;


%% Gains
KP_APz = 3;
KI_APz = 0*0.1044;
KD_APz = 3;

KP_APtheta = 3;
KI_APtheta = 0*0.1466;
KD_APtheta = 3;

KP_APpsi = 3;
KI_APpsi = 0;
KD_APpsi = 12.199;








%% Autopilot (depth)
zerr = z_ref - z;
zerrint = zerr*Ts+zerr_int_prev;
zerrdot = (zerr-zerr_prev)/Ts;
dvz = KP_APz*zerr+KI_APz*zerrint+KD_APz*zerrdot;

theta_ref = 0;
thetaerr = (theta_ref - theta)*180/pi;
thetaerrint = thetaerr*Ts+thetaerr_int_prev;
thetaerrdot = (thetaerr-thetaerr_prev)/Ts;
dvtheta = KP_APtheta*thetaerr+KI_APtheta*thetaerrint+KD_APtheta*thetaerrdot;

dv = dvz + dvtheta;

%% Autopilot (yaw)
psierr = (psi_ref - psi)*180/pi;
psierrint = psierr*Ts+psierr_int_prev;
psierrdot = (psierr-psierr_prev)/Ts;
dh = KP_APpsi*psierr+KI_APpsi*psierrint+KD_APpsi*psierrdot;


%% Control Allocation
d1 = -dv+dh; 
d2 = -dv-dh; 
d3 = dv-dh; 
d4 = dv+dh; 
d5 = dv; 
dX = [d1 ; d2 ; d3 ; d4 ; d5];





%% Save variables for next loop
zerr_prev = zerr;
zerr_int_prev = zerrint;
thetaerr_prev = thetaerr;
thetaerr_int_prev = thetaerrint;
psierr_prev = psierr;
psierr_int_prev = psierrint;

== matlab function ctrl_TT/Controller/FF velocity ctrl ==
  settings: updateMethod=DISCRETE
  data: v_ref input; n output
function n   = fcn(v_ref)




KP_n = 5;
FF_inv = 4;



%% Prop
n = v_ref/FF_inv;

== matlab function ctrl_TT/HDM/HDM B3/Effective Veloicity Calclation/MATLAB Function ==
  data: nh input; n1 input; aX output; n2 input; n3 input; n4 input; nB input; urX1 input; urX2 input; urX3 input; urX4 input; urXB input; UeX output
function [aX,UeX] = fcn(nh,n1,n2,n3,n4,nB,urX1,urX2,urX3,urX4,urXB)

%urXi: relative velocity of rigid body motion and wave particle velocity to the ith stern plane
%ni  : base vector of i-th plane's axis direction
%nh  : base vector of the hull axis direction
IP=zeros(5,1); %IP determines the sign of the angle of attack. if the dot product is negative, angle is greater than 90degs.
aX=zeros(5,1);

np1=dot(nh,urX1)*nh+dot(n1,urX1)*n1;
np2=dot(nh,urX2)*nh+dot(n2,urX2)*n2;
np3=dot(nh,urX3)*nh+dot(n3,urX3)*n3;
np4=dot(nh,urX4)*nh+dot(n4,urX4)*n4;
npB=dot(nh,urXB)*nh+dot(nB,urXB)*nB;

arg1=dot(np1,urX1)/(norm(np1)*norm(urX1));
arg2=dot(np2,urX2)/(norm(np2)*norm(urX2));
arg3=dot(np3,urX3)/(norm(np3)*norm(urX3));
arg4=dot(np4,urX4)/(norm(np4)*norm(urX4));
arg5=dot(npB,urXB)/(norm(npB)*norm(urXB));

%to prevent numerical error: acos returns complex solution. used if statement
if arg1 >=1
   aX(1,1)=0;
else
   aX(1,1)=acos(arg1)*180/pi*sqrt(2);
end

if arg2 >=1
   aX(2,1)=0;
else
   aX(2,1)=acos(arg2)*180/pi*sqrt(2);
end

if arg3 >=1
   aX(3,1)=0;
else
   aX(3,1)=acos(arg3)*180/pi*sqrt(2);
end

if arg4 >=1
   aX(4,1)=0;
else
   aX(4,1)=acos(arg4)*180/pi*sqrt(2);
end

if arg5 >=1
   aX(5,1)=0;
else
   aX(5,1)=acos(arg5)*180/pi;
end

d1=cross(n1,nh);
d2=cross(n2,nh);
d3=cross(n3,nh);
d4=cross(n4,nh);
dB=cross(nB,nh);

IP(1,1)=dot(d1,urX1);
IP(2,1)=dot(d2,urX2);
IP(3,1)=dot(d3,urX3);
IP(4,1)=dot(d4,urX4);
IP(5,1)=dot(dB,urXB);

for i=1:5
    if IP(i,1)<0
        aX(i,1)=-aX(i,1)
    end
end    

UeX=[norm(urX1); norm(urX2); norm(urX3); norm(urX4); norm(urXB);];
end

== matlab function ctrl_TT/HDM/HDM B3/Effective Veloicity Calclation/MATLAB Function1 ==
  data: rX1 input; urX1 output; rX2 input; urX2 output; urX3 output; urX4 output; urXB output; rX3 input; rX4 input; rXB input; U_ship input
function [urX1,urX2,urX3,urX4,urXB]= fcn(rX1,rX2,rX3,rX4,rXB,U_ship)

%rXi: position vector of Stern planes from the CG
%rXB: position vector of sail planes from the CG
%U_ship: rigid body velcity in the ship system

u_ship=[U_ship(1); U_ship(2); U_ship(3);]
w_ship=[U_ship(4); U_ship(5); U_ship(6);]

urX1=-u_ship+cross(rX1,w_ship);
urX2=-u_ship+cross(rX2,w_ship);
urX3=-u_ship+cross(rX3,w_ship);
urX4=-u_ship+cross(rX4,w_ship);
urXB=-u_ship+cross(rXB,w_ship);

end

== matlab function ctrl_TT/HDM/HDM B3/Effective Veloicity Calclation/MATLAB Function2 ==
  data: Bv input; alpha output; beta output; Umag output; uCG input; vCG input; wCG input
function [alpha,beta,Umag] = fcn(Bv,uCG,vCG,wCG)

    u_eff=uCG-Bv(1);
    v_eff=vCG-Bv(2);
    w_eff=wCG-Bv(3);
    
    U_eff=[u_eff; v_eff; w_eff;];
    
    if abs(u_eff) <= 1e-8
        alpha=90; beta=90;
        if v_eff < 0
            beta = -90;
        end
        if w_eff < 0
            alpha = -90;
        end
    else
        beta  = -atan(v_eff/u_eff)*180/pi;
        alpha =  atan(w_eff/u_eff)*180/pi;
    end
    
    Umag =norm(U_eff);
end

== matlab function ctrl_TT/HDM/HDM B3/K/Mx ==
  data: Bx input; Bv input; Ba input; CKup input; CKur input; CKpp input; CKuvw input; Umag input; UeX input; dLCG input; dmass input; CNdXi input; K output; KApp output; K_hull output; Xg parameter; Bb parameter; Xb parameter; Mb parameter; Zg parameter; Zb parameter; Kh_total output; Kpp output; Kprop output; Kvm input; KAppAll output; BFK input; KStat output; Qprop input
function [K,KApp,K_hull,Kh_total,Kpp,Kprop,KAppAll,KStat]  = fcn(Bx,Bv,Ba, CKup,CKur,CKpp,CKuvw,Umag,UeX,dLCG,dmass,CNdXi,Xg,Bb,Xb,Mb,Zg,Zb,Kvm,BFK,Qprop)
%Bx,Bv,Ba are the body motion position, velocity, acceleration in ship coordinate
%Wv,Wa are the wave particle velocity, acceleration in ship coordinate

u=Bv(1); v=Bv(2); w=Bv(3); p=Bv(4); q=Bv(5); r=Bv(6);
x=Bx(1); y=Bx(2); z=Bx(3); phi=Bx(4); theta=Bx(5); psi=Bx(6);
a1=Ba(1); a2=Ba(2); a3=Ba(3); a4=Ba(4); a5=Ba(5); a6=Ba(6); 

KdX1=70.2^3*1025*CNdXi(1)*UeX(1)^2;
KdX2=70.2^3*1025*CNdXi(2)*UeX(2)^2;
KdX3=70.2^3*1025*CNdXi(3)*UeX(3)^2;
KdX4=70.2^3*1025*CNdXi(4)*UeX(4)^2;

Kup = -70.2^3*1025*(-2.9648E-04*u*p)*u^2;
Kur = 70.2^3*1025*(-5.6192E-05*u*r)*u^2;
Kpp = 70.2^3*1025*(-1.0622E-01*p*abs(p));
Kuvw=0.5*70.2^3*1025*CKuvw*Umag^2;
Kprop=Qprop;

KAppAll=[KdX1; KdX2; KdX3; KdX4;];

K_hull=Kuvw+Kup+Kur+Kpp;
KApp=KdX1+KdX2+KdX3+KdX4;
KStat= (Xg*(Mb+dmass))*cos(theta)*sin(phi)+BFK;%(Xg*(Mb+dmass)-Xb*Bb)*cos(theta)*sin(phi);
Kh_total=K_hull+KApp+KStat+Kpp+Kprop;
K=K_hull+KApp+KStat+Kvm+Kpp+Kprop;
end

== matlab function ctrl_TT/HDM/HDM B3/M/My ==
  data: Bx input; Bv input; Ba input; Mqq input; Mwq input; Mprop input; Muvw input; Umag input; UeSP input; dLCG input; dmass input; MdXi input size=5; MY output; Xg parameter; Bb parameter; Xb parameter; Mb parameter; Zg parameter; Zb parameter; Mvm input; MYApp output; MYStat output; Mprop output; M_hull output; MY_hyd output; MYApp_All output; BFM input
function [MY, MYApp, MYStat, Mprop, M_hull,MY_hyd,MYApp_All] = fcn(Bx,Bv,Ba,Mqq,Mwq,Mprop,Muvw,Umag,UeSP,dLCG,dmass,MdXi,Xg,Bb,Xb,Mb,Zg,Zb,Mvm,BFM)
%wqfunction [MY,MYApp,MYStat,Mprop,M_hull]  = fcn(Bx,Bv,Ba,Mqq,Mwq,Muq,Mprop,Muvw,Umag,UeSP,dLCG,dmass,MdXi,Xg,Bb,Xb,Mb,Zg,Zb,Mvm,M_ext)
%Bx,Bv,Ba are the body motion position, velocity, acceleration in ship coordinate
%Wv,Wa are the wave particle velocity, acceleration in ship coordinate

u=Bv(1); v=Bv(2); w=Bv(3); p=Bv(4); q=Bv(5); r=Bv(6);
x=Bx(1); y=Bx(2); z=Bx(3); phi=Bx(4); theta=Bx(5); psi=Bx(6);
a1=Ba(1); a2=Ba(2); a3=Ba(3); a4=Ba(4); a5=Ba(5); a6=Ba(6); 

%MYuq=0.5*70.2^4*1025*Muq
%MYStat=Bb*9.81*dLCG*cos(theta)-Bb*9.81*(Zb-Zg)*sin(theta);

MYX1=0.5*70.2^3*1025*MdXi(1)*UeSP(1)^2;
MYX2=0.5*70.2^3*1025*MdXi(2)*UeSP(2)^2;
MYX3=0.5*70.2^3*1025*MdXi(3)*UeSP(3)^2;
MYX4=0.5*70.2^3*1025*MdXi(4)*UeSP(4)^2;
MYXb=0.5*70.2^3*1025*MdXi(5)*UeSP(5)^2;

MYApp_All=[MYX1; MYX2; MYX3; MYX4; MYXb;];

MYStat= BFM;
MYqq=0.5*70.2^5*1025*Mqq*q*abs(q);
MYuq=0.5*70.2^4*1025*u*q*1.9444E-03*1.1;

MYwq=0.5*70.2^4*1025*Mwq*w*abs(q);
MYuvw=0.5*70.2^3*1025*(Muvw)*Umag^2;
MYApp=(MYX1+MYX2+MYX3+MYX4+MYXb)*1;
Mprop=-1025*70.2^4*u*q*Mprop;

M_hull=MYuvw+MYuq;
MY_hyd=MYApp+MYStat+Mprop+M_hull;
MY=MYApp+MYStat+Mprop+M_hull+Mvm;
end

== matlab function ctrl_TT/HDM/HDM B3/N/Mz ==
  data: Bx input; Bv input; Ba input; CNr input; CNrr input; CNvr input; CNuvw input; Umag input; UeX input; dLCG input; dmass input; CNdXi input; N output; NApp output; N_hull output; Xg parameter; Bb parameter; Xb parameter; Mb parameter; Zg parameter; Zb parameter; Nh_Total output; Nprop output; NStat output; Nvm input; BFN input
function [N,NApp,N_hull,Nh_Total,Nprop,NStat]  = fcn(Bx,Bv,Ba, CNr,CNrr,CNvr,CNuvw,Umag,UeX,dLCG,dmass,CNdXi,Xg,Bb,Xb,Mb,Zg,Zb,Nvm,BFN)
%Bx,Bv,Ba are the body motion position, velocity, acceleration in ship coordinate
%Wv,Wa are the wave particle velocity, acceleration in ship coordinate

u=Bv(1); v=Bv(2); w=Bv(3); p=Bv(4); q=Bv(5); r=Bv(6);
x=Bx(1); y=Bx(2); z=Bx(3); phi=Bx(4); theta=Bx(5); psi=Bx(6);
a1=Ba(1); a2=Ba(2); a3=Ba(3); a4=Ba(4); a5=Ba(5); a6=Ba(6); 

NdX1=70.2^3*1025*CNdXi(1)*UeX(1)^2;
NdX2=70.2^3*1025*CNdXi(2)*UeX(2)^2;
NdX3=70.2^3*1025*CNdXi(3)*UeX(3)^2;
NdX4=70.2^3*1025*CNdXi(4)*UeX(4)^2;

Nr  =0.5*70.2^3*1025*(7.6545E-03*0.8*u*r)*u^2*0.5;
%Nr  =-0.5*70.2^3*1025*CNr*u^2*3;
Nvr =0.5*70.2^3*1025*CNvr*u^2; %major source of error in it
Nrr =-0.5*70.2^3*1025*CNrr*r^2*u^2;
Nuvw=0.5*70.2^3*1025*CNuvw*Umag^2;
Nprop=0.5*70.2^3*1025*u^2*(-0.0055*r);

NApp=NdX1+NdX2+NdX3+NdX4;
N_hull=Nuvw+Nr+Nvr+Nrr;
NHullVM=N_hull+Nvm;
NStat= BFN;

Nh_Total=N_hull+NApp+NStat;

N=N_hull+NApp+NStat+Nvm;
end

== matlab function ctrl_TT/HDM/HDM B3/Thrust & Torque/Tprop ==
  data: speed input; Td input; Tprop output; n_0 input; Qprop output
function [Tprop,Qprop]   = fcn(speed,Td,n_0)
J=speed/(n_0*5);
Kt=-0.0923*J^2-0.3652*J+0.4786;
Kq=-2.1064E-02*J^2 - 3.2470E-02*J + 6.3982E-02;
Tprop=Kt*(1-Td)*(1025*n_0^2*5^4);
Qprop=Kq*1025*n_0^2*5^5

== matlab function ctrl_TT/HDM/HDM B3/Wave, Virtual Mass and Hydrostatic/MATLAB Function ==
  data: Rs input; cvm input; Awrs input; Fvm output; Mvm output
function [Fvm,Mvm]  = fcn(Rs,cvm,Awrs)
%Inputs to the subroutine
%Rs  = position vector of sectional elements' CG in ship coordinate system.
%dm  = water volume mass of each section. could be replaced by the sectional volume.
%Ars = acceleration vector of each section in ship coordinate system
%Aws = sectional acceleration vector of wave particles in ship coordinate system
%cvm = sectional virtual mass coefficients. Input size is n x 3.

%Outputs from the subroutine
%Fvm  = total virtual mass force vector
%dFvm = sectional virtual mass force vector
%Mvm  = total virtual mass moment vector
%dMvm = sectional virtual mass moment vector

ni=15;%length(cvm); %number of sectional elements
dFvm = zeros(ni,3); dMvm = zeros(ni,3);
 Fvm = zeros(1,3);   Mvm = zeros(1,3);
 
 dXm=zeros(ni,1);
 dYm=zeros(ni,1);
 dZm=zeros(ni,1);
 dKm=zeros(ni,1);
 dMm=zeros(ni,1);
 dNm=zeros(ni,1);
 
%Fvm_out  = zeros(3);  Mvm_out = zeros(3); %temporary variable for report

for i=1:ni
    for j=1:3
        dFvm(i,j) = cvm(i,j)*Awrs(i,j);    
         Fvm(1,j)   = Fvm(1,j)+dFvm(i,j);   
    end
    
    Rsi   = [Rs(i,1);     Rs(i,2);   Rs(i,3);];
    dFvmi = [dFvm(i,1); dFvm(i,2); dFvm(i,3);];
    dMvmi = cross(Rsi,dFvmi);%cross(dFvmi,Rsi);
    
    for j=1:3
        dMvm(i,j) = dMvmi(j);
         Mvm(1,j) = Mvm(1,j)+dMvm(i,j);
    end
    
    for i=1:ni
        dXm(i,1)=dFvm(i,1);
        dYm(i,1)=dFvm(i,2);
        dZm(i,1)=dFvm(i,3);
        dKm(i,1)=dMvm(i,1);
        dMm(i,1)=dMvm(i,2);
        dNm(i,1)=dMvm(i,3);    
    end

  end
